simulink model "lab7"  (Simulink 7.5)
settings: Solver=ode3  StartTime=0.0  StopTime=10.0  RelTol=1e-3
libraries: simulink x1
settings Model: Creator=Dranik_win  LastModifiedBy=Dranik_win

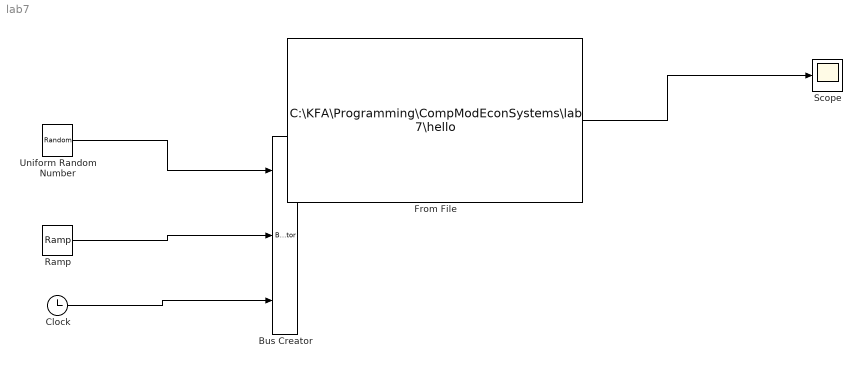
== system lab7 ==
  Bus Creator : BusCreator  Inputs=3
  Clock : Clock
      settings: Decimation=10
  From File : FromFile  FileName=C:\KFA\Programming\CompModEconSystems\lab 7\hello  SampleTime=0
  Ramp : simulink/Sources/Ramp  SystemSampleTime=-1  slope=1  start=0  X0=0
  Scope : Scope
  Uniform Random Number : UniformRandomNumber  SampleTime=0.1
  wires:
  Ramp/1 -> Bus Creator/2
  Uniform Random Number/1 -> Bus Creator/1
  Clock/1 -> Bus Creator/3
  From File/1 -> Scope/1
